simulink model "SingleTrackSimulation_R2016b"  (R2018b)
settings: Solver=VariableStepAuto  StartTime=0.0  StopTime=10.0  RelTol=1e-3
values from neighbouring files (symbols this model uses):
  a = 1    [SingleTrack.m]    (also in simulatedPlot.m)
  b = 1    [SingleTrack.m]    (also in simulatedPlot.m)
  C = 50    [SingleTrack.m]
  delta_r_option = 3    [SingleTrack.m]
  Iz = 5    [SingleTrack.m]
  speed = 2    [SingleTrack.m]
undefined symbols (not defined in the file or in its folder): sigbuilder_block, steering_factor
settings Model: Creator=Knoll  LastModifiedBy=Knoll
settings CodeAppCC: StateflowObjectComments=on

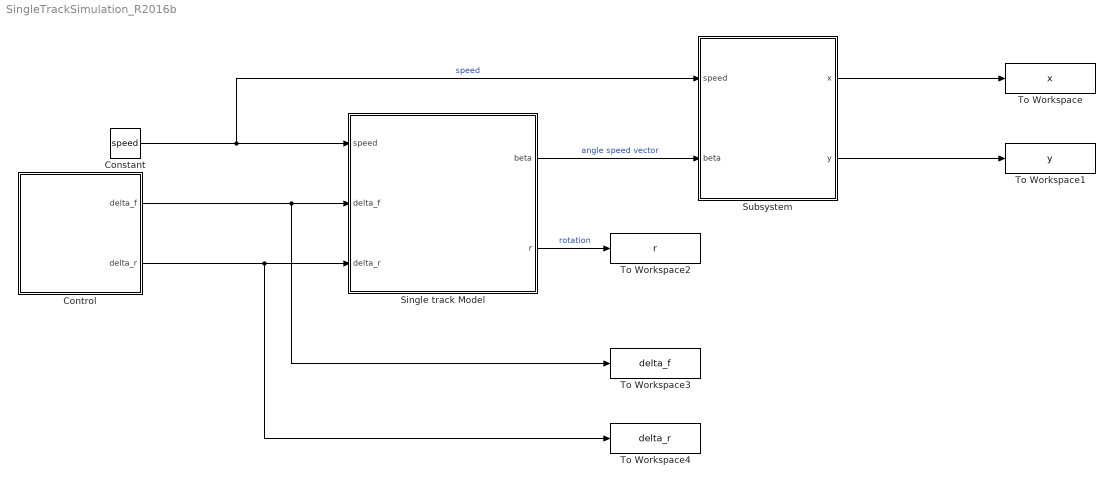
== system SingleTrackSimulation_R2016b ==
  Constant : Constant  Value=speed
  Control : Subsystem
      mask Display: image('C:\Users\Knoll\Dropbox\Studium\Seminararbeit\Matlab\Single_Track\Images\controller.png');
  Single track Model : Subsystem  mask{m=20, a=a, b=b, Iz=Iz}
      mask Display: image('C:\Users\Knoll\Dropbox\Studium\Seminararbeit\Matlab\Single_Track\Images\images.png'); % Use "Edit Image" on toolstrip to change.
  Subsystem : Subsystem
      mask Display: image('C:\Users\Knoll\Dropbox\Studium\Seminararbeit\Matlab\Single_Track\Images\convert-photo-to-icon-8.png');
  To Workspace : ToWorkspace  VariableName=x  SaveFormat=Timeseries  SampleTime=-1
  To Workspace1 : ToWorkspace  VariableName=y  SaveFormat=Timeseries  SampleTime=-1
  To Workspace2 : ToWorkspace  VariableName=r  SaveFormat=Timeseries  SampleTime=-1
  To Workspace3 : ToWorkspace  VariableName=delta_f  SaveFormat=Timeseries  SampleTime=-1
  To Workspace4 : ToWorkspace  VariableName=delta_r  SaveFormat=Timeseries  SampleTime=-1
  wires:
  Subsystem/2(y) -> To Workspace1/1
  Constant/1 -> Subsystem/1(speed), Single track Model/1(speed)  "speed"
  Subsystem/1(x) -> To Workspace/1
  Single track Model/2(r) -> To Workspace2/1  "rotation"
  Control/2(delta_r) -> To Workspace4/1, Single track Model/3(delta_r)
  Control/1(delta_f) -> Single track Model/2(delta_f), To Workspace3/1
  Single track Model/1(beta) -> Subsystem/2(beta)  "angle speed vector"

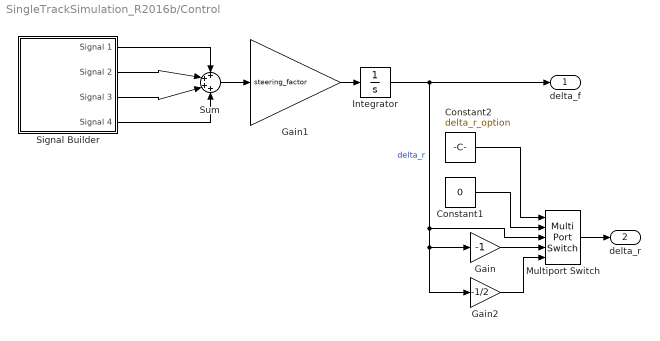
== system SingleTrackSimulation_R2016b/Control ==
  Constant1 : Constant  Value=0
  Constant2 : Constant  Value=delta_r_option
  Gain : Gain  Gain=-1
  Gain1 : Gain  Gain=steering_factor
  Gain2 : Gain  Gain=-1/2
  Integrator : Integrator
  Multiport Switch : MultiPortSwitch  Inputs=4
  Signal Builder : Subsystem  Tag=STV Subsys  LoadFcn=sigbuilder_block('load');  StartFcn=sigbuilder_block('start');  StopFcn=sigbuilder_block('stop');  ClipboardFcn=sigbuilder_block('clipboard');  mask(Sigbuilder block){tuvar=[0:10]}
      mask help: Simulink:masks:SigbuilderBlock_MD
      mask init:
      | if ~strcmp(get_param(bdroot(gcbh),'SimulationStatus'),'stopped') tuvar = sigbuilder_block('maskInit'); end
      settings: CopyFcn=sigbuilder_block('copy');  DeleteFcn=sigbuilder_block('delete');  ModelCloseFcn=sigbuilder_block('modelClose');  PreSaveFcn=sigbuilder_block('preSave');  PauseFcn=sigbuilder_block('pause');  ContinueFcn=sigbuilder_block('continue');  NameChangeFcn=sigbuilder_block('namechange');  OpenFcn=sigbuilder_block('open',[437.6 199.2 550.4 400 ]);  CloseFcn=sigbuilder_block('close');
      mask Display: plot(0, 0, 100, 100,[2, 2, 32, 32, 2], [68, 8, 8, 68, 68],[32, 2], [38, 38], [32, 19, 2],[53, 60, 44], [32, 17, 17, 2],[16, 16, 31, 31]);txt = getActiveGroup(gcbh);text(2, 100, txt,'verticalAlignment', 'top');
  Sum : Sum  Inputs=++++
  delta_f : Outport
  delta_r : Outport  Port=2
  wires:
  Integrator/1 -> delta_f/1, Gain2/1, Gain/1, Multiport Switch/3  "delta_r"
  Constant1/1 -> Multiport Switch/2
  Gain/1 -> Multiport Switch/4
  Multiport Switch/1 -> delta_r/1
  Constant2/1 -> Multiport Switch/1
  Signal Builder/1(Signal 1) -> Sum/1
  Signal Builder/2(Signal 2) -> Sum/2
  Signal Builder/3(Signal 3) -> Sum/3
  Signal Builder/4(Signal 4) -> Sum/4
  Gain1/1 -> Integrator/1
  Sum/1 -> Gain1/1
  Gain2/1 -> Multiport Switch/5

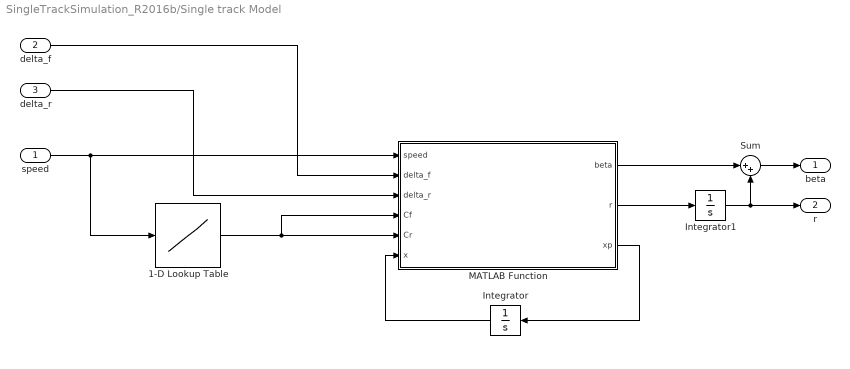
== system SingleTrackSimulation_R2016b/Single track Model ==
  speed : Inport
  delta_f : Inport  Port=2
  delta_r : Inport  Port=3
  1-D Lookup Table : Lookup_n-D  NumberOfTableDimensions=1  BreakpointsForDimension1=[-5:5]  Table=C* ones(1, 11)  InternalRulePriority=Speed  RndMeth=Simplest  InputSameDT=on
  Integrator : Integrator  InitialCondition=[0;0]
  Integrator1 : Integrator
  MATLAB Function : MATLAB Function  TreatAsAtomicUnit=on
  Sum : Sum  Inputs=|++
  beta : Outport
  r : Outport  Port=2
  wires:
  Integrator/1 -> MATLAB Function/6(x)
  delta_r/1 -> MATLAB Function/3(delta_r)
  MATLAB Function/3(xp) -> Integrator/1
  delta_f/1 -> MATLAB Function/2(delta_f)
  speed/1 -> 1-D Lookup Table/1, MATLAB Function/1(speed)
  1-D Lookup Table/1 -> MATLAB Function/4(Cf), MATLAB Function/5(Cr)
  Integrator1/1 -> Sum/2, r/1
  MATLAB Function/2(r) -> Integrator1/1
  MATLAB Function/1(beta) -> Sum/1
  Sum/1 -> beta/1

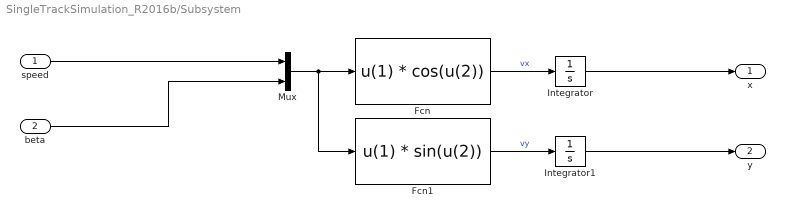
== system SingleTrackSimulation_R2016b/Subsystem ==
  speed : Inport
  beta : Inport  Port=2
  Fcn : Fcn  Expr=u(1) * cos(u(2))
  Fcn1 : Fcn  Expr=u(1) * sin(u(2))
  Integrator : Integrator
  Integrator1 : Integrator
  Mux : Mux  Inputs=2
  x : Outport
  y : Outport  Port=2
  wires:
  Integrator/1 -> x/1
  Fcn1/1 -> Integrator1/1  "vy"
  Fcn/1 -> Integrator/1  "vx"
  Integrator1/1 -> y/1
  speed/1 -> Mux/1
  Mux/1 -> Fcn1/1, Fcn/1
  beta/1 -> Mux/2

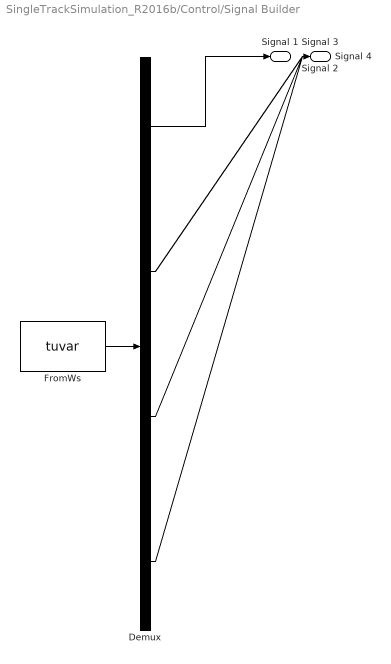
== system SingleTrackSimulation_R2016b/Control/Signal Builder ==
  Demux : Demux  Tag=STV Demux
  FromWs : FromWorkspace  Tag=STV FromWs  VariableName=tuvar  SampleTime=0
      SigBuilderData=|
      | common.afterFinalStr = 'Extrapolate'
      | common.sampleTime = 0
      | dataSet.timeRange = [0 10]
      | dataSet.name = 'Group 1'
      | sbobj.Groups.Name = 'Group 1'
      | sbobj.Groups.Signals(1).Name = 'Signal 1'
      | sbobj.Groups.Signals(1).XData = [0 1 1 2 2 10]
      | sbobj.Groups.Signals(1).YData = [0 0 1 1 0 0]
      | sbobj.Groups.Signals(2).Name = 'Signal 2'
      | sbobj.Groups.Signals(2).XData = [0 3 3 4 4 10]
      | sbobj.Groups.Signals(2).YData = [0 0 -1 -1 0 0]
      | sbobj.Groups.Signals(3).Name = 'Signal 3'
      | sbobj.Groups.Signals(3).XData = [0 5 5 6 6 10]
      | sbobj.Groups.Signals(3).YData = [0 0 -1 -1 0 0]
      | sbobj.Groups.Signals(4).Name = 'Signal 4'
      | sbobj.Groups.Signals(4).XData = [0 7 7 8 8 10]
      | sbobj.Groups.Signals(4).YData = [0 0 1 1 0 0]
  Signal 1 : Outport  Tag=STV Outport
  Signal 2 : Outport  Tag=STV Outport  Port=2
  Signal 3 : Outport  Tag=STV Outport  Port=3
  Signal 4 : Outport  Tag=STV Outport  Port=4
  wires:
  Demux/1 -> Signal 1/1
  FromWs/1 -> Demux/1
  Demux/2 -> Signal 2/1
  Demux/3 -> Signal 3/1
  Demux/4 -> Signal 4/1

== matlab function SingleTrackSimulation_R2016b/Single track Model/MATLAB Function ==
  data: beta output; r output; speed input; delta_f input; delta_r input; Cf input; Cr input; x input; xp output; m parameter; a parameter; b parameter; Iz parameter
function [beta, r, xp] = singleTrackModel(speed, delta_f, delta_r, Cf, Cr, x, m, a, b, Iz)

m= 1;
A = [-(Cf + Cr)/(m*speed), (-1-((a * Cf - b*Cr)/(m*speed^2)));
     -(a*Cf - b*Cr)/Iz, -((a^2*Cf + b^2*Cr) / (Iz*speed))];
 
B = [Cf/(m*speed), Cr/(m*speed);
     (a*Cf)/Iz, (-b*Cr)/Iz];
 
u = [delta_f; 
     delta_r];
 
xp = zeros(2, 1); 
xp = A*x + B*u;

r = x(2);
beta = x(1);
